simulink model "punto1"  (Simulink 5.0)
settings: Solver=ode45  StartTime=0.0  StopTime=100.0  RelTol=1e-3
settings Model: LastModifiedBy=Juan

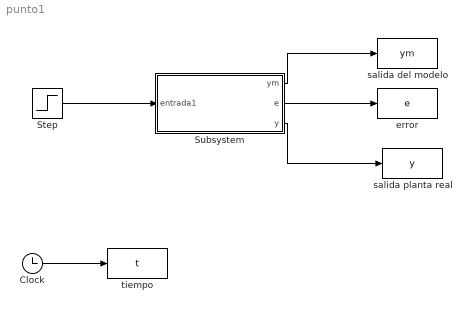
== system punto1 ==
  Clock : Clock
      settings: Decimation=10
  Step : Step  SampleTime=0
  Subsystem : Subsystem  mask{am=1, bm=1, a=1, b=1, kp=1, km=2, gama=0.1, g=1}
      mask prompts: am "a del modelo (am)"; bm "b del modelo (bm)"; a "a de la planta real (a)"; b "b de la planta real (b)"; kp "ganancia de la planta real (kp)"; km "ganancia del modelo (km)"; g "constante g"
      mask init:
      | a=1;
      | b=1;
      mask Display: disp('Sistema')
  error : ToWorkspace  VariableName=e  SampleTime=-1  SaveFormat=Array
  salida del modelo : ToWorkspace  VariableName=ym  SampleTime=-1  SaveFormat=Array
  salida planta real : ToWorkspace  VariableName=y  SampleTime=-1  SaveFormat=Array
  tiempo : ToWorkspace  VariableName=t  SampleTime=-1  SaveFormat=Array
  wires:
  Clock/1 -> tiempo/1
  Subsystem/1(ym) -> salida del modelo/1
  Step/1 -> Subsystem/1(entrada1)
  Subsystem/2(e) -> error/1
  Subsystem/3(y) -> salida planta real/1

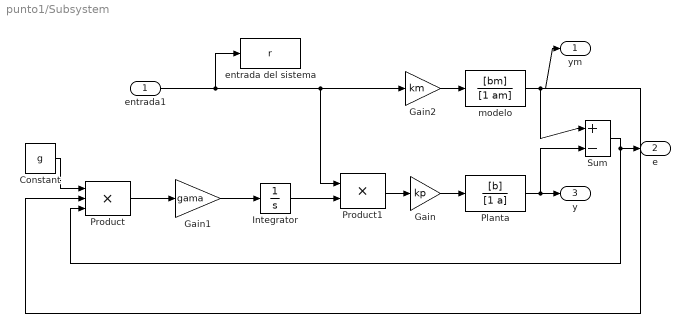
== system punto1/Subsystem ==
  entrada1 : Inport
  Constant : Constant  Value=g
  Gain : Gain  Gain=kp  SaturateOnIntegerOverflow=on
  Gain1 : Gain  Gain=gama  SaturateOnIntegerOverflow=on
  Gain2 : Gain  Gain=km  SaturateOnIntegerOverflow=on
  Integrator : Integrator
  Planta : TransferFcn  Numerator=[b]  Denominator=[1 a]
  Product : Product  Inputs=3  SaturateOnIntegerOverflow=on
  Product1 : Product  SaturateOnIntegerOverflow=on
  Sum : Sum  Inputs=|+-  SaturateOnIntegerOverflow=on
  entrada del sistema : ToWorkspace  VariableName=r  SampleTime=-1  SaveFormat=Array
  modelo : TransferFcn  Numerator=[bm]  Denominator=[1 am]
  ym : Outport
  e : Outport  Port=2
  y : Outport  Port=3
  wires:
  Product/1 -> Gain1/1
  modelo/1 -> Sum/1, Product/2, ym/1
  Planta/1 -> Sum/2, y/1
  Product1/1 -> Gain/1
  Integrator/1 -> Product1/2
  Gain1/1 -> Integrator/1
  Sum/1 -> Product/3, e/1
  Constant/1 -> Product/1
  Gain2/1 -> modelo/1
  Gain/1 -> Planta/1
  entrada1/1 -> entrada del sistema/1, Product1/1, Gain2/1
